simulink model "TCMSSystem"  (R2019b)
settings: configuration reference "ConfigSet_TCMSSystem_Reference" (kept outside this file)
model workspace (MAT data in the model file):
  Prm_TCMSSystem : Simulink.Parameter (value not decoded)
  SampleTime = 0.05
symbols that are objects in the model workspace (value not decoded): Prm_TCMSSystem
undefined symbols (not defined in the file): ADDIntervention, AK1Status, AK2Status, AKContactorStatus, AllDoorsClosed, AllLeftDoorsClosed, AllRightDoorsClosed, APS1Fault, APS1Isolated, APS1OutputVoltage, APS1Status, APS2Fault, APS2Isolated, APS2OutputVoltage, APS2Status, APSKAKContactor, ASCOEnd1, ASCOEnd2, ATBMode, ATCBypassMode, ATCStatusNotOK, ATOMode, ATPLowSpeedCutoutStatus, ATPMode, AuxCompressor, BatteryCurrent, BatteryIsolationContactor, BatteryTemperature, BatteryVoltage, BCG1Fault, BCG1Isolated, BCG1IsolationFailed, BCG1OutputCurrent, BCG1Status, BCG2Fault, BCG2Isolated, BCG2OutputCurrent, BCG2Status, BCGOutputVoltage, BECU1AxleLockedWheelSet1, BECU2AxleLockedWheelSet2, BECUFaulty, BECUMajorFault, BECUMinorFault, BECUStatus, BIC1Inside, BIC1Outside, BIC2Inside, BIC2Outside, Bogie, Bogie1WSPStatus, Bogie2WSPStatus, BogieFaulty, BogieIsolationStatus, BogieSupportedMass, BrakeCylinderPressureGauge, BrakeLoopCBTripped, BrakeLoopOpenTL, BrakeTrainLineStatus, BrakingDemand ... (+215)
libraries: TimersLib x257, simulink x137, LatchesLib x42, VectorOperationsLib x15, TestBenchLib x12, MathOperationsLib x2, FiltersLib x1
(part 16 of 16)

== system TCMSSystem/TCMSSystemPerVehicle/EnabledTCMSVehicle/TCMSTractionBraking/TractionBrakingControl/CabControlsExtract/Speed Limit Protection/50kphConditions ==
  note: Conditions for 50 Kph
      | 2 bogies isolated due to any of the isolation cocks
  <Bogie> : Inport
  PneumaticTrainSum : Inport  Port=2
  TractionBrakingBogieData : Inport  Port=3
  2_Bogies_Isolated : simulink/Logic and Bit Operations/Compare To Constant  relop=>=  const=2  OutDataTypeStr=boolean
  Bus Selector1 : BusSelector  OutputSignals=NoOfBogieIsolated
  For Each Subsystem : Subsystem  TreatAsAtomicUnit=on
  Logical Operator1 : Logic  Operator=OR  Inputs=1  AllPortsSameDT=off  OutDataTypeStr=boolean
  NOT : Logic  Operator=NOT  AllPortsSameDT=off  OutDataTypeStr=boolean
  OR1 : Logic  Operator=OR  Inputs=3  AllPortsSameDT=off  OutDataTypeStr=boolean
  OR2 : Logic  Operator=OR  Inputs=1  AllPortsSameDT=off  OutDataTypeStr=boolean
  Subsystem : Subsystem
  True : Outport
  wires:
  2_Bogies_Isolated/1 -> OR1/2
  Bus Selector1/1 -> 2_Bogies_Isolated/1  "<NoOfBogieIsolated>"
  PneumaticTrainSum/1 -> Bus Selector1/1
  OR1/1 -> True/1
  Subsystem/1(<AirSuspensionBogie1Deflated>) -> OR2/1
  <Bogie>/1 -> Subsystem/1(In1)
  OR2/1 -> OR1/1
  For Each Subsystem/1(Out1) -> Logical Operator1/1
  Logical Operator1/1 -> NOT/1
  NOT/1 -> OR1/3
  TractionBrakingBogieData/1 -> For Each Subsystem/1(In1)

== system TCMSSystem/TCMSSystemPerVehicle/EnabledTCMSVehicle/TCMSTractionBraking/TractionBrakingControl/CabControlsExtract/Speed Limit Protection/Special Modes Case ==
  note: SH 26Sept24
      | This speed limit logic needs to be more simplified, but in the interest of time, adding this Speed Restriction signal.
      | Earlier, the flag indicating the train speed exceeding the speed limit would work ONLY when the speed limit value was NOT 0.
      | But this caused a problem when we need to restrict the train movement when the speed limit is actually 0.
      | Hence added this extra input for no train movement to be authorized.
  note: Special Modes Overspeed:
      | Both in SCS and Wash Mode, TCMS applies FSB.
      |
      | Special Limit Active:
      | In SCS, Powering is not available once 23kmph speed is
      | reached and becomes available once speed falls below 17kmph.
      |
      | In Wash Mode, Powering is not available once 3kmph speed is
      | reached and becomes available once speed falls below 2kmph.
  note: In wash mode, for example, for 3KMPH set point, traction will be cut at 3 kmph,
      | 50% FSB shall be applied at 4 KMPH, and FSB shall be applied at 5 KMPH.
      | This logic is extended for 4 and 5 KMPH set points.
  CBTCIn : Inport
  WashModeActive : Inport  Port=2
  <Speedometer> : Inport  Port=3
  SpeedLimit : Inport  Port=4
  IOControls : Inport  Port=5
  In Bus Element : Inport  Port=6  PortName=DisplayControl  Element=ATPLowModeActivated
  In Bus Element1 : Inport  Port=6  PortName=DisplayControl  Element=ShuntModeActivated
  In Bus Element2 : Inport  Port=6  PortName=DisplayControl  Element=ShuntModeMinSpeed
  SpeedRestrict : Inport  Port=7
  Bus Selector1 : BusSelector  OutputSignals=ATCBypassState
  Bus Selector3 : BusSelector  OutputSignals=ModeSelector
  Constant : Constant  Value=0
  Data Type Conversion{,1,3..6} (6 alike) : DataTypeConversion
  If : If  NumInputs=6  IfExpression=u1>0 & u2 == 0 & u3>0  ElseIfExpressions=u2 > 0, u1>0 & u2 == 0 & u4>0, u5>0, u6>0  ShowElse=off
  If Action Subsystem : Subsystem  TreatAsAtomicUnit=on
  If Action Subsystem1 : Subsystem  TreatAsAtomicUnit=on
  If Action Subsystem2 : Subsystem  TreatAsAtomicUnit=on
  "LowSpeedCutoutMode " : Subsystem  TreatAsAtomicUnit=on
  Merge : Merge  Inputs=5
  Merge1 : Merge  Inputs=5
  OR : Logic  Operator=OR  Inputs=3  AllPortsSameDT=off  OutDataTypeStr=boolean
  RMF : simulink/Logic and Bit Operations/Compare To Constant  relop===  const=3  OutDataTypeStr=boolean
  RMR : simulink/Logic and Bit Operations/Compare To Constant  relop===  const=1  OutDataTypeStr=boolean
  Relational Operator1 : RelationalOperator  OutDataTypeStr=boolean  RndMeth=Simplest
  "ShuntModeActive " : Subsystem  TreatAsAtomicUnit=on
  Switch : Switch  Criteria=u2 > Threshold
  kphTomps10 : Gain  Gain=1/3.6
  SpecialModesOverspeed : Outport
  SpecialLimitActive : Outport  Port=2
  wires:
  Merge/1 -> Data Type Conversion3/1  "SpecialCaseOvSpd"
  CBTCIn/1 -> Bus Selector1/1
  Bus Selector1/1 -> Data Type Conversion/1  "<ATCBypassState>"
  WashModeActive/1 -> Data Type Conversion1/1  "WashModeActive"
  If/1 -> If Action Subsystem/Action  "SCS_Forward"
  If/2 -> If Action Subsystem1/Action  "Washmode"
  If Action Subsystem/1(Ovspd) -> Merge/1
  If Action Subsystem1/1(OvSpd) -> Merge/2
  <Speedometer>/1 -> Relational Operator1/1, "LowSpeedCutoutMode "/1(Spd), If Action Subsystem2/1(Spd), If Action Subsystem/1(Spd), If Action Subsystem1/1(Spd), "ShuntModeActive "/1(Spd)  "Speedometer"
  Data Type Conversion/1 -> If/1
  Data Type Conversion1/1 -> If/2
  Data Type Conversion4/1 -> SpecialLimitActive/1
  Data Type Conversion3/1 -> SpecialModesOverspeed/1
  RMR/1 -> Data Type Conversion6/1  "Reverse"
  Merge1/1 -> OR/1  "SpecialCaseSpeedLimit"
  If/3 -> If Action Subsystem2/Action  "SCS_Reverse"
  IOControls/1 -> Bus Selector3/1
  Bus Selector3/1 -> RMF/1, RMR/1  "<ModeSelector>"
  RMF/1 -> Data Type Conversion5/1  "Forward"
  Data Type Conversion5/1 -> If/3
  Data Type Conversion6/1 -> If/4
  If Action Subsystem/2(Limit) -> Merge1/1
  If Action Subsystem2/2(Limit) -> Merge1/3
  If Action Subsystem1/2(Limit) -> Merge1/2
  If Action Subsystem2/1(Ovspd) -> Merge/3
  SpeedLimit/1 -> Relational Operator1/2, If Action Subsystem1/2(WMLim), "ShuntModeActive "/2(MaxSpd), "LowSpeedCutoutMode "/2(MaxSpd), Switch/2
  OR/1 -> Data Type Conversion4/1
  If/4 -> "ShuntModeActive "/Action  "ShuntModeActive"
  If/5 -> "LowSpeedCutoutMode "/Action  "LowSpeedCutoutMode"
  In Bus Element1/1 -> If/5
  In Bus Element/1 -> If/6
  "LowSpeedCutoutMode "/2(Limit) -> Merge1/5
  "ShuntModeActive "/2(Limit) -> Merge1/4
  "ShuntModeActive "/1(OvSpd) -> Merge/4
  "LowSpeedCutoutMode "/1(Ovspd) -> Merge/5
  In Bus Element2/1 -> kphTomps10/1
  kphTomps10/1 -> "ShuntModeActive "/3(MinSpd)
  Switch/1 -> OR/2
  Relational Operator1/1 -> Switch/1
  Constant/1 -> Switch/3
  SpeedRestrict/1 -> OR/3

== system TCMSSystem/TCMSSystemPerVehicle/EnabledTCMSVehicle/TCMSTractionBraking/TractionBrakingControl/CabControlsExtract/TractionBrakingRefCalc/HBRelease ==
  note: Timer ON delay makes sure that
      | the traction demand stays constant
      |  for a significant time to avoid the
      | unintensional holding brakes release.
      | Especially in ATO/UTO mode where the Traction demand is generated by error between the permitted speed and actual speed.
  TractionForceFB : Inport
  NotImmobilise : Inport  Port=2
  ATO/UTO : Inport  Port=3
  HBStatus : Inport  Port=4
  Abs : Abs
  Compare To Constant : simulink/Logic and Bit Operations/Compare To Constant  relop=>  const=1000  OutDataTypeStr=boolean
  Constant1 : Constant  Value=0
  Constant3 : Constant
  Display : Display
  First Order Low Pass Filter : FiltersLib/First Order Low Pass Filter  FilterSpecificationSource=internal  FilterSpecificationType=Specify Time Constant  FilterSpecificationValue=0.01  SampleTime=-1
      settings: SourceProductName=Filters
  Switch : Switch  Criteria=u2 > Threshold
  Switch1 : Switch  Criteria=u2 > Threshold
  Switch3 : Switch  Criteria=u2 > Threshold
  TimerOnDelay NoInit : TimersLib/TimerOnDelay NoInit  UpperSaturationLimit=1  OutputTime=off  SampleTime=-1
      settings: SourceProductName=Sydac Utilities
  HBRelease : Outport
  wires:
  Switch/1 -> HBRelease/1
  Switch3/1 -> Switch/1
  Constant1/1 -> Switch3/3
  ATO/UTO/1 -> Switch/2
  NotImmobilise/1 -> Switch3/2
  Compare To Constant/1 -> TimerOnDelay NoInit/1
  Constant3/1 -> Switch1/3
  Switch1/1 -> Switch3/1
  HBStatus/1 -> Switch1/2
  TimerOnDelay NoInit/1 -> Switch/3, Switch1/1
  TractionForceFB/1 -> Abs/1
  Abs/1 -> First Order Low Pass Filter/1, Compare To Constant/1
  First Order Low Pass Filter/1 -> Display/1

== system TCMSSystem/TCMSSystemPerVehicle/EnabledTCMSVehicle/TCMSTractionBraking/TractionBrakingControl/CabControlsExtract/TractionBrakingRefCalc/HoldingBrake ==
  note: TractionCommand's range is 0 to 100
      | BrakingCommand's range is 0 to 100
  note: Emergency Traction Mode:
      | Holding brake apply condition is simply listed as train speed being < 1km/h.
      | The reset priority latch allows for release when applying traction.
  note: Holding brake applies 70% service brake
  BrakingCommand : Inport
  VehicleSpeed : Inport  Port=2
  TCMSHoldingBrakeRelease : Inport  Port=3
  AND1 : Logic  AllPortsSameDT=off  OutDataTypeStr=boolean
  Abs : Abs
  Compare To Constant : simulink/Logic and Bit Operations/Compare To Constant  relop=<=  const=0.5  OutDataTypeStr=boolean
  Compare To Zero : simulink/Logic and Bit Operations/Compare To Zero  relop=>  OutDataTypeStr=boolean
  Compare To Zero1 : simulink/Logic and Bit Operations/Compare To Zero  relop===  OutDataTypeStr=boolean
  Data Type Conversion : DataTypeConversion
  Detect Increase : simulink/Logic and Bit Operations/Detect Increase  vinit=0.0  OutDataTypeStr=boolean
  HBDemand : Constant  Value=70
  NoHBDemand : Constant  Value=0
  OR : Logic  Operator=OR  AllPortsSameDT=off  OutDataTypeStr=boolean
  SR Latch - Reset Priority : LatchesLib/SR Latch - Reset Priority  initial_condition=0
      settings: SourceProductName=Latches
  Switch3 : Switch  Criteria=u2 > Threshold
  HoldingBrakeDemand : Outport
  HoldingBrakeApplied : Outport  Port=2
  wires:
  BrakingCommand/1 -> Compare To Zero1/1, Compare To Zero/1
  SR Latch - Reset Priority/1 -> Data Type Conversion/1, Switch3/2  "HBApply"
  TCMSHoldingBrakeRelease/1 -> SR Latch - Reset Priority/2  "HoldingBrakeRelease"
  VehicleSpeed/1 -> Abs/1
  AND1/1 -> SR Latch - Reset Priority/1  "HoldingBrakeApply"
  HBDemand/1 -> Switch3/1
  Switch3/1 -> HoldingBrakeDemand/1
  NoHBDemand/1 -> Switch3/3
  Compare To Zero/1 -> OR/1
  Data Type Conversion/1 -> HoldingBrakeApplied/1
  OR/1 -> AND1/2
  Detect Increase/1 -> OR/2
  Compare To Zero1/1 -> Detect Increase/1
  Compare To Constant/1 -> AND1/1
  Abs/1 -> Compare To Constant/1

== system TCMSSystem/TCMSSystemPerVehicle/EnabledTCMSVehicle/TCMSTractionBraking/TractionBrakingControl/CabControlsExtract/TractionBrakingRefCalc/TBRefDemandFromCBTC ==
  CBTC : Inport
  Abs : Abs
  Bus Selector2 : BusSelector  OutputSignals=ATOTBDemandPct,ATOTraction,ATOBraking,NoServiceBrakeOrder,DriverModeSelection,NotImmobilise
  Compare To Constant : simulink/Logic and Bit Operations/Compare To Constant  relop=>=  const=5  OutDataTypeStr=boolean
  Product : Product
  Product1 : Product
  ATO/UTOModeActive : Outport
  RefTraction : Outport  Port=2
  RefBraking : Outport  Port=3
  NoSB : Outport  Port=4
  NotImmobilise : Outport  Port=5
  wires:
  Bus Selector2/5 -> Compare To Constant/1  "<DriverModeSelection>"
  CBTC/1 -> Bus Selector2/1
  Compare To Constant/1 -> ATO/UTOModeActive/1
  Bus Selector2/4 -> NoSB/1  "<NoServiceBrakeOrder>"
  Bus Selector2/6 -> NotImmobilise/1  "<NotImmobilise>"
  Bus Selector2/2 -> Product1/2  "<ATOTraction>"
  Bus Selector2/1 -> Abs/1  "<ATOTBDemandPct>"
  Abs/1 -> Product/1, Product1/1
  Product1/1 -> RefTraction/1
  Bus Selector2/3 -> Product/2  "<ATOBraking>"
  Product/1 -> RefBraking/1

== system TCMSSystem/TCMSSystemPerVehicle/EnabledTCMSVehicle/TCMSTractionBraking/TractionBrakingDisplay/OperatingandOtherScreen/CabUnitDisplay/CabActiveUnitDisplay ==
  In Bus Element4 : Inport  PortName=ElectricalSignals  Element=ForwardDirection
  In Bus Element5 : Inport  PortName=ElectricalSignals  Element=ReverseDirection
  In Bus Element6 : Inport  PortName=ElectricalSignals  Element=TractionOn
  In Bus Element7 : Inport  PortName=ElectricalSignals  Element=BrakeOn
  In Bus Element8 : Inport  PortName=ElectricalSignals  Element=TractionSafe
  In Bus Element3 : Inport  PortName=ElectricalSignals  Element=Speedometer
  In Bus Element14 : Inport  PortName=ElectricalSignals  Element=ZeroSpeed
  In Bus Element : Inport  Port=2  PortName=TractionUnitData  Element=TractiveEffortAchieved
  In Bus Element1 : Inport  Port=2  PortName=TractionUnitData  Element=EDBrakingEffortAchieved
  In Bus Element2 : Inport  Port=2  PortName=TractionUnitData  Element=TractiveEffortPossible
  In Bus Element9 : Inport  Port=2  PortName=TractionUnitData  Element=EDBrakingEffortPossible
  In Bus Element10 : Inport  Port=2  PortName=TractionUnitData  Element=TractivePowerAchieved
  In Bus Element11 : Inport  Port=2  PortName=TractionUnitData  Element=EDBrakingPowerAchieved
  In Bus Element12 : Inport  Port=2  PortName=TractionUnitData  Element=TractivePowerPossible
  In Bus Element13 : Inport  Port=2  PortName=TractionUnitData  Element=EDBrakingPowerPossible
  Action Port : ActionPort  ActionPortLabel=if(u1 > 0)
  Bus Creator : BusCreator  Inputs=15
  Data Type Conversion{,1..14} (15 alike) : DataTypeConversion  OutDataTypeStr=double
  Out1 : Outport
  wires:
  Data Type Conversion2/1 -> Bus Creator/5  "TractionOn"
  Data Type Conversion1/1 -> Bus Creator/2  "ReverseDirection"
  Data Type Conversion/1 -> Bus Creator/1  "ForwardDirection"
  Bus Creator/1 -> Out1/1
  In Bus Element4/1 -> Data Type Conversion/1
  In Bus Element5/1 -> Data Type Conversion1/1
  In Bus Element6/1 -> Data Type Conversion2/1
  In Bus Element/1 -> Data Type Conversion5/1
  In Bus Element8/1 -> Data Type Conversion4/1
  In Bus Element7/1 -> Data Type Conversion3/1
  Data Type Conversion3/1 -> Bus Creator/6  "BrakeOn"
  Data Type Conversion4/1 -> Bus Creator/7  "TractionSafe"
  Data Type Conversion5/1 -> Bus Creator/8  "UnitTractiveEffortAchieved"
  Data Type Conversion11/1 -> Bus Creator/14  "UnitTractivePowerPossible"
  Data Type Conversion10/1 -> Bus Creator/13  "UnitEDBrakingPowerAchieved"
  Data Type Conversion9/1 -> Bus Creator/12  "UnitTractivePowerAchieved"
  In Bus Element10/1 -> Data Type Conversion9/1
  In Bus Element11/1 -> Data Type Conversion10/1
  In Bus Element12/1 -> Data Type Conversion11/1
  In Bus Element9/1 -> Data Type Conversion8/1
  In Bus Element2/1 -> Data Type Conversion7/1
  In Bus Element1/1 -> Data Type Conversion6/1
  Data Type Conversion6/1 -> Bus Creator/9  "UnitEDBrakingEffortAchieved"
  Data Type Conversion7/1 -> Bus Creator/10  "UnitTractiveEffortPossible"
  Data Type Conversion8/1 -> Bus Creator/11  "UnitEDBrakingEffortPossible"
  In Bus Element13/1 -> Data Type Conversion12/1
  Data Type Conversion12/1 -> Bus Creator/15  "UnitEDBrakingPowerPossible"
  In Bus Element14/1 -> Data Type Conversion14/1
  In Bus Element3/1 -> Data Type Conversion13/1
  Data Type Conversion13/1 -> Bus Creator/3  "Speedometer"
  Data Type Conversion14/1 -> Bus Creator/4  "ZeroSpeed"

== system TCMSSystem/TCMSSystemPerVehicle/EnabledTCMSVehicle/TCMSTractionBraking/TractionBrakingDisplay/OperatingandOtherScreen/CabUnitDisplay/CabInactiveNoDisplay ==
  Action Port : ActionPort  ActionPortLabel=else
  Bus Creator1 : BusCreator  Inputs=15
  Constant{1..15} (15 alike) : Constant  Value=0
  Out1 : Outport
  wires:
  Bus Creator1/1 -> Out1/1
  Constant8/1 -> Bus Creator1/8  "UnitTractiveEffortAchieved"
  Constant6/1 -> Bus Creator1/6  "BrakeOn"
  Constant7/1 -> Bus Creator1/7  "TractionSafe"
  Constant3/1 -> Bus Creator1/1  "ForwardDirection"
  Constant4/1 -> Bus Creator1/2  "ReverseDirection"
  Constant10/1 -> Bus Creator1/10  "UnitTractiveEffortPossible"
  Constant14/1 -> Bus Creator1/13  "UnitEDBrakingPowerAchieved"
  Constant15/1 -> Bus Creator1/14  "UnitTractivePowerPossible"
  Constant12/1 -> Bus Creator1/11  "UnitEDBrakingEffortPossible"
  Constant9/1 -> Bus Creator1/9  "UnitEDBrakingEffortAchieved"
  Constant13/1 -> Bus Creator1/12  "UnitTractivePowerAchieved"
  Constant5/1 -> Bus Creator1/5  "TractionOn"
  Constant11/1 -> Bus Creator1/15  "UnitEDBrakingPowerPossible"
  Constant2/1 -> Bus Creator1/4  "ZeroSpeed"
  Constant1/1 -> Bus Creator1/3  "Speedometer"

== system TCMSSystem/TCMSSystemPerVehicle/LimpHomeTCMSVehicle/TCMSTractionBraking/TractionBrakingControl/CabControlsExtract/Speed Limit Protection/0kphConditions ==
  note: Conditions for 0 Kph
      | Direction Switch at Standby/Off
  PneumaticTrainSum : Inport
  6_Bogies_Isolated : simulink/Logic and Bit Operations/Compare To Constant  relop=>=  const=6  OutDataTypeStr=boolean
  Bus Selector1 : BusSelector  OutputSignals=NoOfBogieIsolated
  True : Outport
  wires:
  PneumaticTrainSum/1 -> Bus Selector1/1
  Bus Selector1/1 -> 6_Bogies_Isolated/1  "<NoOfBogieIsolated>"
  6_Bogies_Isolated/1 -> True/1

== system TCMSSystem/TCMSSystemPerVehicle/LimpHomeTCMSVehicle/TCMSTractionBraking/TractionBrakingControl/CabControlsExtract/Speed Limit Protection/10kphConditions ==
  note: Conditions for 10 Kph
      | Restricted Reverse Mode
  CBTCIn : Inport
  Bus Selector2 : BusSelector  OutputSignals=DriverModeSelection
  Logical Operator : Logic  Operator=OR  Inputs=1  AllPortsSameDT=off  OutDataTypeStr=boolean
  RMR : simulink/Logic and Bit Operations/Compare To Constant  relop===  const=3  OutDataTypeStr=boolean
  True : Outport
  wires:
  Bus Selector2/1 -> RMR/1  "<DriverModeSelection>"
  CBTCIn/1 -> Bus Selector2/1
  RMR/1 -> Logical Operator/1  "RMR"
  Logical Operator/1 -> True/1

== system TCMSSystem/TCMSSystemPerVehicle/LimpHomeTCMSVehicle/TCMSTractionBraking/TractionBrakingControl/CabControlsExtract/Speed Limit Protection/TCMSDisplaySpeedLim ==
  note: Condition
      | Diplayed limit KMPH
      |
      | Off
      | 0
      |
      | Standby
      | 0
      |
      | RMR
      | 10
  IOControl : Inport
  Bus Selector1 : BusSelector  OutputSignals=ModeSelector
  Constant : Constant  Value=0
  Constant1 : Constant  Value=25
  Constant2 : Constant  Value=10
  OR2 : Logic  Operator=OR  AllPortsSameDT=off  OutDataTypeStr=boolean
  OffPosition : simulink/Logic and Bit Operations/Compare To Constant  relop===  const=0  OutDataTypeStr=boolean
  RMRPosition : simulink/Logic and Bit Operations/Compare To Constant  relop===  const=1  OutDataTypeStr=boolean
  StandbyPosition : simulink/Logic and Bit Operations/Compare To Constant  relop===  const=2  OutDataTypeStr=boolean
  Switch : Switch  Criteria=u2 > Threshold
  Switch2 : Switch  Criteria=u2 > Threshold
  kphTomps1 : Gain  Gain=1/3.6
  kphTomps4 : Gain  Gain=1/3.6
  TCMSSpeedLimit : Outport
  wires:
  OffPosition/1 -> OR2/1
  Bus Selector1/1 -> StandbyPosition/1, RMRPosition/1, OffPosition/1  "<ModeSelector>"
  IOControl/1 -> Bus Selector1/1
  OR2/1 -> Switch/2  "ZeroLimit"
  StandbyPosition/1 -> OR2/2
  Constant/1 -> Switch/1
  Constant1/1 -> kphTomps1/1
  Switch2/1 -> Switch/3
  Constant2/1 -> kphTomps4/1
  RMRPosition/1 -> Switch2/2
  Switch/1 -> TCMSSpeedLimit/1
  kphTomps4/1 -> Switch2/1
  kphTomps1/1 -> Switch2/3

== system TCMSSystem/TCMSSystemPerVehicle/LimpHomeTCMSVehicle/TCMSTractionBraking/TractionBrakingControl/CabControlsExtract/TractionBrakingRefCalc/HBRelease ==
  TractionRef : Inport
  Compare To Constant : simulink/Logic and Bit Operations/Compare To Constant  relop=>  const=10  OutDataTypeStr=boolean
  HBRelease : Outport
  wires:
  Compare To Constant/1 -> HBRelease/1
  TractionRef/1 -> Compare To Constant/1

== system TCMSSystem/TCMSSystemPerVehicle/LimpHomeTCMSVehicle/TCMSTractionBraking/TractionBrakingControl/CabControlsExtract/TractionBrakingRefCalc/HoldingBrake ==
  note: Emergency Traction Mode:
      | Holding brake apply condition is simply listed as train speed being < 1km/h.
      | The reset priority latch allows for release when applying traction.
  note: Holding brake applies 70% service brake
  TractionCmd : Inport
  ZeroSpeed : Inport  Port=2
  TCMSHoldingBrakeRelease : Inport  Port=3
  AND1 : Logic  AllPortsSameDT=off  OutDataTypeStr=boolean
  AND2 : Logic  AllPortsSameDT=off  OutDataTypeStr=boolean
  Compare To Zero : simulink/Logic and Bit Operations/Compare To Zero  relop=<=  OutDataTypeStr=boolean
  Data Type Conversion : DataTypeConversion
  HBDemand : Constant  Value=70
  NoHBDemand : Constant  Value=0
  SR Latch - Reset Priority : LatchesLib/SR Latch - Reset Priority  initial_condition=0
      settings: SourceProductName=Latches
  Switch3 : Switch  Criteria=u2 > Threshold
  Unit Delay : UnitDelay  SampleTime=-1  HasFrameUpgradeWarning=on
  HoldingBrakeDemand : Outport
  HoldingBrakeApplied : Outport  Port=2
  wires:
  TractionCmd/1 -> Compare To Zero/1
  SR Latch - Reset Priority/1 -> Data Type Conversion/1, Switch3/2, Unit Delay/1  "HBApply"
  TCMSHoldingBrakeRelease/1 -> AND2/1  "HoldingBrakeRelease"
  ZeroSpeed/1 -> AND1/1
  AND1/1 -> SR Latch - Reset Priority/1  "HoldingBrakeApply"
  HBDemand/1 -> Switch3/1
  Switch3/1 -> HoldingBrakeDemand/1
  NoHBDemand/1 -> Switch3/3
  Compare To Zero/1 -> AND1/2
  Unit Delay/1 -> AND2/2
  AND2/1 -> SR Latch - Reset Priority/2  "HoldingBrakeRelease"
  Data Type Conversion/1 -> HoldingBrakeApplied/1

== system TCMSSystem/TCMSSystemPerVehicle/EnabledTCMSVehicle/TCMSTractionBraking/TractionBrakingControl/CabControlsExtract/Speed Limit Protection/40kphConditions/For Each Subsystem ==
  In1 : Inport  Partition=on  PartitionDimension=1  PartitionWidth=1  PartitionOffset=0
  Speedometer : Inport  Port=2
  Bus Selector2 : BusSelector  OutputSignals=TCUSlipDetected
  For Each : ForEach  DisableCoverage=on
  SR Latch - Reset Priority : LatchesLib/SR Latch - Reset Priority  initial_condition=0
      settings: SourceProductName=Latches
  Stop : simulink/Logic and Bit Operations/Compare To Constant  relop=<  const=0.05  OutDataTypeStr=boolean
  Out2 : Outport  ConcatenationDimension=1
  wires:
  In1/1 -> Bus Selector2/1
  Bus Selector2/1 -> SR Latch - Reset Priority/1  "<TCUSlipDetected>"
  Speedometer/1 -> Stop/1
  Stop/1 -> SR Latch - Reset Priority/2
  SR Latch - Reset Priority/1 -> Out2/1

== system TCMSSystem/TCMSSystemPerVehicle/EnabledTCMSVehicle/TCMSTractionBraking/TractionBrakingControl/CabControlsExtract/Speed Limit Protection/40kphConditions/Subsystem ==
  In1 : Inport  Partition=on  PartitionDimension=1  PartitionWidth=1  PartitionOffset=0
  Bus Selector2 : BusSelector  OutputSignals=BECU1LoadPressureLow
  For Each : ForEach  DisableCoverage=on
  <BECU1LoadPressureLow> : Outport  ConcatenationDimension=1
  wires:
  Bus Selector2/1 -> <BECU1LoadPressureLow>/1  "<BECU1LoadPressureLow>"
  In1/1 -> Bus Selector2/1

== system TCMSSystem/TCMSSystemPerVehicle/EnabledTCMSVehicle/TCMSTractionBraking/TractionBrakingControl/CabControlsExtract/Speed Limit Protection/50kphConditions/For Each Subsystem ==
  In1 : Inport  Partition=on  PartitionDimension=1  PartitionWidth=1  PartitionOffset=0
  Bus Selector2 : BusSelector  OutputSignals=EDBrakeNotIsolated
  For Each : ForEach  DisableCoverage=on
  Out1 : Outport  ConcatenationDimension=1
  wires:
  In1/1 -> Bus Selector2/1
  Bus Selector2/1 -> Out1/1  "<EDBrakeNotIsolated>"

== system TCMSSystem/TCMSSystemPerVehicle/EnabledTCMSVehicle/TCMSTractionBraking/TractionBrakingControl/CabControlsExtract/Speed Limit Protection/50kphConditions/Subsystem ==
  In1 : Inport  Partition=on  PartitionDimension=1  PartitionWidth=1  PartitionOffset=0
  Bus Selector2 : BusSelector  OutputSignals=AirSuspensionBogie1Deflated
  For Each : ForEach  DisableCoverage=on
  <AirSuspensionBogie1Deflated> : Outport  ConcatenationDimension=1
  wires:
  Bus Selector2/1 -> <AirSuspensionBogie1Deflated>/1  "<AirSuspensionBogie1Deflated>"
  In1/1 -> Bus Selector2/1

== system TCMSSystem/TCMSSystemPerVehicle/EnabledTCMSVehicle/TCMSTractionBraking/TractionBrakingControl/CabControlsExtract/Speed Limit Protection/Special Modes Case/If Action Subsystem ==
  Spd : Inport
  Action Port : ActionPort  ActionPortLabel=if(u1>0 & u2 == 0 & u3>0)
  Constant3 : Constant  Value=25/3.6
  Data Type Conversion : DataTypeConversion
  Relational Operator1 : RelationalOperator  Operator=>  OutDataTypeStr=boolean  RndMeth=Simplest
  Relay : Relay  OnSwitchValue=25/3.6  OffSwitchValue=15/3.6
  Ovspd : Outport
  Limit : Outport  Port=2
  wires:
  Spd/1 -> Relay/1, Relational Operator1/1
  Constant3/1 -> Relational Operator1/2
  Relational Operator1/1 -> Data Type Conversion/1  "SCSOverspeed"
  Data Type Conversion/1 -> Ovspd/1
  Relay/1 -> Limit/1  "SCSLimit"

== system TCMSSystem/TCMSSystemPerVehicle/EnabledTCMSVehicle/TCMSTractionBraking/TractionBrakingControl/CabControlsExtract/Speed Limit Protection/Special Modes Case/If Action Subsystem1 ==
  Spd : Inport
  WMLim : Inport  Port=2
  Action Port : ActionPort  ActionPortLabel=elseif(u2 > 0)
  Bias : Bias  Bias=0.278
  Bias1 : Bias  Bias=0.278
  Bias2 : Bias  Bias=0.278
  Bias3 : Bias  Bias=-0.278
  Constant : Constant
  Constant1 : Constant  Value=2
  Constant2 : Constant  Value=0
  Data Type Conversion : DataTypeConversion
  Data Type Conversion1 : DataTypeConversion
  Relational Operator : RelationalOperator  Operator=>  OutDataTypeStr=boolean  RndMeth=Simplest
  Relational Operator1 : RelationalOperator  OutDataTypeStr=boolean  RndMeth=Simplest
  Relational Operator2 : RelationalOperator  OutDataTypeStr=boolean  RndMeth=Simplest
  Relational Operator3 : RelationalOperator  OutDataTypeStr=boolean  RndMeth=Simplest
  SR Latch - Set Priority : LatchesLib/SR Latch - Set Priority  initial_condition=0
      settings: SourceProductName=Latches
  Switch : Switch  Criteria=u2 > Threshold
  Switch1 : Switch  Criteria=u2 > Threshold
  OvSpd : Outport
  Limit : Outport  Port=2
  wires:
  Switch/1 -> Data Type Conversion/1  "WashModeOverspeed"
  Bias/1 -> Relational Operator1/2
  Relational Operator1/1 -> Switch1/2  "WashModeOverspeed"
  Bias1/1 -> Bias2/1
  Bias2/1 -> Relational Operator2/2
  Switch1/1 -> Switch/3  "WashModeOverspeed"
  Relational Operator2/1 -> Switch/2  "WashModeOverspeed"
  Constant/1 -> Switch/1
  Constant1/1 -> Switch1/1
  Constant2/1 -> Switch1/3
  Data Type Conversion/1 -> OvSpd/1
  Relational Operator3/1 -> SR Latch - Set Priority/2  "WashModeLimit"
  Relational Operator/1 -> SR Latch - Set Priority/1  "WashModeLimit"
  Bias3/1 -> Relational Operator3/2
  WMLim/1 -> Relational Operator/2, Bias3/1, Bias1/1, Bias/1
  SR Latch - Set Priority/1 -> Data Type Conversion1/1
  Spd/1 -> Relational Operator3/1, Relational Operator/1, Relational Operator1/1, Relational Operator2/1
  Data Type Conversion1/1 -> Limit/1

== system TCMSSystem/TCMSSystemPerVehicle/EnabledTCMSVehicle/TCMSTractionBraking/TractionBrakingControl/CabControlsExtract/Speed Limit Protection/Special Modes Case/If Action Subsystem2 ==
  Spd : Inport
  Action Port : ActionPort  ActionPortLabel=elseif( u1>0 & u2 == 0 & u4>0)
  Constant3 : Constant  Value=10/3.6
  Data Type Conversion : DataTypeConversion
  Relational Operator1 : RelationalOperator  Operator=>  OutDataTypeStr=boolean  RndMeth=Simplest
  Relay1 : Relay  OnSwitchValue=10/3.6  OffSwitchValue=2/3.6
  Ovspd : Outport
  Limit : Outport  Port=2
  wires:
  Relay1/1 -> Limit/1  "RMRLimit"
  Spd/1 -> Relational Operator1/1, Relay1/1
  Constant3/1 -> Relational Operator1/2
  Relational Operator1/1 -> Data Type Conversion/1  "RMROverspeed"
  Data Type Conversion/1 -> Ovspd/1

== system TCMSSystem/TCMSSystemPerVehicle/EnabledTCMSVehicle/TCMSTractionBraking/TractionBrakingControl/CabControlsExtract/Speed Limit Protection/Special Modes Case/LowSpeedCutoutMode  ==
  Spd : Inport
  MaxSpd : Inport  Port=2
  Action Port : ActionPort  ActionPortLabel=elseif( u6>0)
  Constant3 : Constant  Value=2/3.6
  Data Type Conversion1 : DataTypeConversion
  Data Type Conversion2 : DataTypeConversion
  Relational Operator : RelationalOperator  Operator=>  OutDataTypeStr=boolean  RndMeth=Simplest
  Relational Operator3 : RelationalOperator  OutDataTypeStr=boolean  RndMeth=Simplest
  Relational Operator4 : RelationalOperator  Operator=<  OutDataTypeStr=boolean  RndMeth=Simplest
  SR Latch - Set Priority : LatchesLib/SR Latch - Set Priority  initial_condition=0
      settings: SourceProductName=Latches
  Ovspd : Outport
  Limit : Outport  Port=2
  wires:
  Relational Operator/1 -> SR Latch - Set Priority/1  "ATPLSCutoutModeUpperLimit"
  Relational Operator4/1 -> SR Latch - Set Priority/2  "ATPLSCutoutModeLowerLimit"
  Data Type Conversion2/1 -> Limit/1
  SR Latch - Set Priority/1 -> Data Type Conversion2/1
  Data Type Conversion1/1 -> Ovspd/1
  MaxSpd/1 -> Relational Operator/2, Relational Operator3/2
  Spd/1 -> Relational Operator4/1, Relational Operator/1, Relational Operator3/1
  Constant3/1 -> Relational Operator4/2
  Relational Operator3/1 -> Data Type Conversion1/1  "ATPLSCutoutModeOverspeed"

== system TCMSSystem/TCMSSystemPerVehicle/EnabledTCMSVehicle/TCMSTractionBraking/TractionBrakingControl/CabControlsExtract/Speed Limit Protection/Special Modes Case/ShuntModeActive  ==
  Spd : Inport
  MaxSpd : Inport  Port=2
  MinSpd : Inport  Port=3
  Action Port : ActionPort  ActionPortLabel=elseif( u5>0)
  Data Type Conversion1 : DataTypeConversion
  Data Type Conversion2 : DataTypeConversion
  Relational Operator : RelationalOperator  Operator=>  OutDataTypeStr=boolean  RndMeth=Simplest
  Relational Operator3 : RelationalOperator  OutDataTypeStr=boolean  RndMeth=Simplest
  Relational Operator4 : RelationalOperator  Operator=<  OutDataTypeStr=boolean  RndMeth=Simplest
  SR Latch - Set Priority : LatchesLib/SR Latch - Set Priority  initial_condition=0
      settings: SourceProductName=Latches
  OvSpd : Outport
  Limit : Outport  Port=2
  wires:
  Spd/1 -> Relational Operator4/1, Relational Operator/1, Relational Operator3/1
  Data Type Conversion1/1 -> OvSpd/1
  SR Latch - Set Priority/1 -> Data Type Conversion2/1
  MinSpd/1 -> Relational Operator4/2
  Data Type Conversion2/1 -> Limit/1
  Relational Operator3/1 -> Data Type Conversion1/1  "ShuntModeOverspeed"
  MaxSpd/1 -> Relational Operator/2, Relational Operator3/2
  Relational Operator/1 -> SR Latch - Set Priority/1  "ShuntModeUpperLimit"
  Relational Operator4/1 -> SR Latch - Set Priority/2  "ShuntModeLowerLimit"

== stateflow chart TCMSSystem/TCMSSystemPerVehicle/EnabledTCMSVehicle/TCMSElectrical/ElectricalControl/Subsystem/Chart ==
  state Init
    en: count=0;
    VCBCloseReq=0;
  state State1
    en: count=count+1;
  state State2
    en: VCBCloseReq=1;
  state State3
    en: VCBCloseReq=0;
  (default) -> Init
  State3 -> Init : [TW_POFF==1]
  Init -> State1 : [TW_TPOR==1]
  State1 -> State2 : [(count==1) & (PantographRaisedFully ==1)]
  State2 -> State3 : [ VCBState==1 ]
  data: TW_TPOR input; TW_POFF input; VCBState input; VCBCloseReq output; count local; PantographRaisedFully input

== matlab function TCMSSystem/TCMSSystemPerVehicle/EnabledTCMSVehicle/OutputsPacking/TCMSDisplayOutputs/TCMSMessageEvents/MessageShortList/TCMS Message Index List/pad ==
  data: u input; y output
function y = find_and_pad(u)
    u1 = find(u);
    y = zeros(10,1);
    for i = 1:length(y);
        if(i <= length(u1) && i <= length(y))
            y(i) = u1(i);
        end
    end
end

== matlab function TCMSSystem/TCMSSystemPerVehicle/EnabledTCMSVehicle/OutputsPacking/TCMSDisplayOutputs/TCMSMessageEvents/MessageShortList/TCMS Message Index List/pad1 ==
  data: u input; y output; y_prev input
function y = persistent_order(u, y_prev)
    y = y_prev;
    %remove any elements from y not in u
    for i=1:length(y)
        if(y(i) > 0 && isempty(find(u == y(i))))
            y(i) = 0;
        end
    end
    %add any new elements from u into y
    for i=1:length(u)
        if(u(i) > 0 && isempty(find(y == u(i)))) %u(i) is not in y
            %find the next empty slot in y
            empty_slots = find(y == 0);
            if(~isempty(empty_slots))
                y(empty_slots(1)) = u(i);
            end
        end
    end
end
